simulink model "heli_v2"  (Simulink 4.00)
settings: Solver=ode45  StartTime=0.0  StopTime=180.0  RelTol=1e-3
settings Model: Creator=stk  LastModifiedBy=shirley  MaxDataPoints=2000000  ExtModeAutoUpdateStatusClock=off

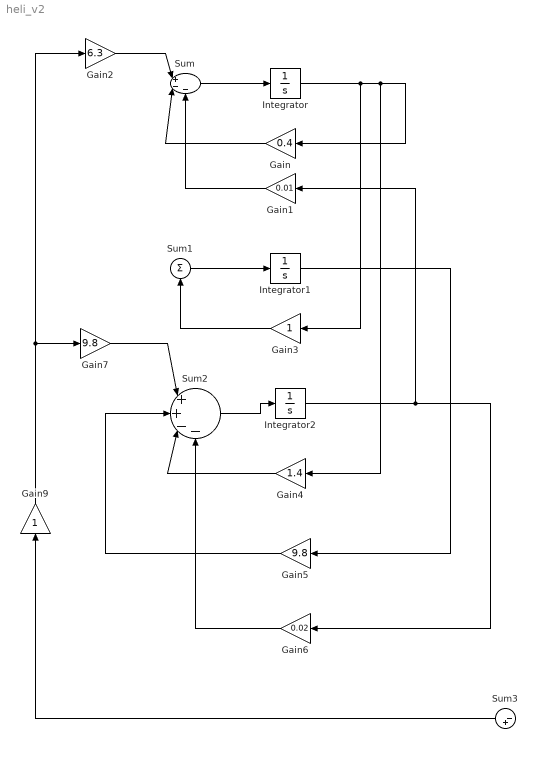
== system heli_v2 ==
  Gain : Gain  Orientation=left  Gain=0.4  Multiplication=Element-wise(K.*u)  SaturateOnIntegerOverflow=on
  Gain1 : Gain  Orientation=left  Gain=0.01  Multiplication=Element-wise(K.*u)  SaturateOnIntegerOverflow=on
  Gain2 : Gain  Gain=6.3  Multiplication=Element-wise(K.*u)  SaturateOnIntegerOverflow=on
  Gain3 : Gain  Orientation=left  Gain=1  Multiplication=Element-wise(K.*u)  SaturateOnIntegerOverflow=on
  Gain4 : Gain  Orientation=left  Gain=1.4  Multiplication=Element-wise(K.*u)  SaturateOnIntegerOverflow=on
  Gain5 : Gain  Orientation=left  Gain=9.8  Multiplication=Element-wise(K.*u)  SaturateOnIntegerOverflow=on
  Gain6 : Gain  Orientation=left  Gain=0.02  Multiplication=Element-wise(K.*u)  SaturateOnIntegerOverflow=on
  Gain7 : Gain  Gain=9.8  Multiplication=Element-wise(K.*u)  SaturateOnIntegerOverflow=on
  Gain9 : Gain  Orientation=up  Gain=1  Multiplication=Element-wise(K.*u)  SaturateOnIntegerOverflow=on
  Integrator : Integrator  ExternalReset=none  InitialConditionSource=internal  InitialCondition=0  LimitOutput=off  UpperSaturationLimit=inf  LowerSaturationLimit=-inf  ShowSaturationPort=off  ShowStatePort=off  AbsoluteTolerance=auto
  Integrator1 : Integrator  ExternalReset=none  InitialConditionSource=internal  InitialCondition=0  LimitOutput=off  UpperSaturationLimit=inf  LowerSaturationLimit=-inf  ShowSaturationPort=off  ShowStatePort=off  AbsoluteTolerance=auto
  Integrator2 : Integrator  ExternalReset=none  InitialConditionSource=internal  InitialCondition=0  LimitOutput=off  UpperSaturationLimit=inf  LowerSaturationLimit=-inf  ShowSaturationPort=off  ShowStatePort=off  AbsoluteTolerance=auto
  Sum : Sum  Inputs=|+--  SaturateOnIntegerOverflow=on
  Sum1 : Sum  Inputs=|+  SaturateOnIntegerOverflow=on
  Sum2 : Sum  Inputs=|++--  SaturateOnIntegerOverflow=on
  Sum3 : Sum  Orientation=left  Inputs=|-+  SaturateOnIntegerOverflow=on
  wires:
  Integrator/1 -> Gain3/1, Gain/1, Gain4/1
  Gain/1 -> Sum/2
  Gain1/1 -> Sum/3
  Sum/1 -> Integrator/1
  Gain2/1 -> Sum/1
  Integrator1/1 -> Gain5/1
  Gain4/1 -> Sum2/3
  Gain5/1 -> Sum2/2
  Gain6/1 -> Sum2/4
  Sum2/1 -> Integrator2/1
  Gain7/1 -> Sum2/1
  Gain9/1 -> Gain2/1, Gain7/1
  ? -> Sum3/2
  Integrator2/1 -> Gain6/1, Gain1/1
  Sum3/1 -> Gain9/1
  Gain3/1 -> Sum1/1
  Sum1/1 -> Integrator1/1
